simulink model "quarter_model_basic_R2019a"  (R2019a)
settings: Solver=VariableStepAuto  StartTime=0.0  StopTime=20  RelTol=1e-3
values from neighbouring files (symbols this model uses):
  b = 1.8*b    (= 3600)    [quarter_model_basic_script.m]    (also in quarter_model_nonlin_script.m = 2000)
  k1 = 1.08e5    (= 108000)    [quarter_model_basic_script.m]    (also in quarter_model_nonlin_script.m)
  k2 = 2.09e4    (= 20900)    [quarter_model_basic_script.m]    (also in quarter_model_nonlin_script.m)
  m1 = 31    [quarter_model_basic_script.m]    (also in quarter_model_nonlin_script.m)
  m2 = 350    [quarter_model_basic_script.m]    (also in quarter_model_nonlin_script.m)
settings Model: Creator=kjartan  LastModifiedBy=kjartan

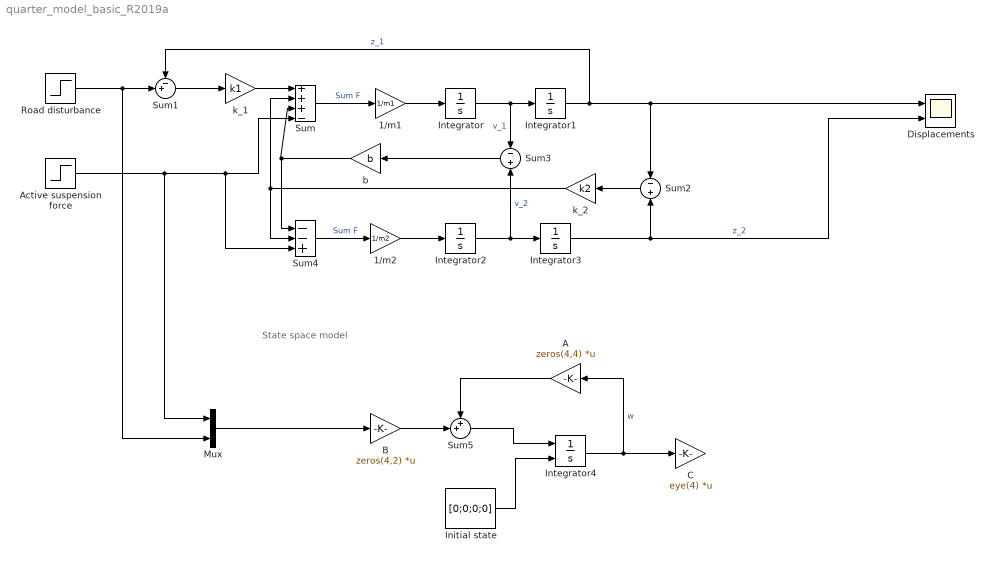
== system quarter_model_basic_R2019a ==
  note: State space model
  1/m1 : Gain  Gain=1/m1
  1/m2 : Gain  Gain=1/m2
  A : Gain  Gain=zeros(4,4)  Multiplication=Matrix(K*u) (u vector)
  Active suspension force : Step  Time=10  After=200  SampleTime=0
  B : Gain  Gain=zeros(4,2)  Multiplication=Matrix(K*u)
  C : Gain  Gain=eye(4)  Multiplication=Matrix(K*u) (u vector)
  Displacements : Scope  NumInputPorts=2
  Initial state : Constant  Value=[0;0;0;0]
  Integrator{,1..3} (4 alike) : Integrator
  Integrator4 : Integrator  InitialConditionSource=external
  Mux : Mux  Inputs=2
  Road disturbance : Step  After=0.1  SampleTime=0
  Sum : Sum  Inputs=+++-
  Sum1 : Sum  Inputs=-+|
  Sum2 : Sum  Inputs=-|+
  Sum3 : Sum  Inputs=-|+
  Sum4 : Sum  Inputs=--+
  Sum5 : Sum  Inputs=++|
  b : Gain  Gain=b
  k_1 : Gain  Gain=k1
  k_2 : Gain  Gain=k2
  wires:
  Integrator/1 -> Sum3/1, Integrator1/1  "v_1"
  Integrator1/1 -> Sum2/1, Displacements/1, Sum1/1  "z_1"
  Integrator2/1 -> Integrator3/1, Sum3/2  "v_2"
  Integrator3/1 -> Sum2/2, Displacements/2  "z_2"
  1/m2/1 -> Integrator2/1
  1/m1/1 -> Integrator/1
  Road disturbance/1 -> Mux/2, Sum1/2
  Sum1/1 -> k_1/1
  Sum3/1 -> b/1
  k_1/1 -> Sum/1
  b/1 -> Sum4/1, Sum/3
  Sum2/1 -> k_2/1
  k_2/1 -> Sum/2, Sum4/2
  Sum/1 -> 1/m1/1  "Sum F"
  Active suspension force/1 -> Mux/1, Sum4/3, Sum/4
  Sum4/1 -> 1/m2/1  "Sum F"
  Initial state/1 -> Integrator4/2
  B/1 -> Sum5/2
  Sum5/1 -> Integrator4/1
  Integrator4/1 -> A/1, C/1  "w"
  A/1 -> Sum5/1
  Mux/1 -> B/1
